simulink model "system13"  (R2019a)
settings: Solver=VariableStepAuto  StartTime=0.0  StopTime=40.0  RelTol=1e-3
values from neighbouring files (symbols this model uses):
  d_y0 = 0    [Lab2.m]
  k2 = sqrt(2*k1)    [Lab2.m]    (also in blockFunc10.m)
  y0 = 0    [Lab2.m]
undefined symbols (not defined in the file or in its folder): sigbuilder_block
settings Model: Creator=Vasco  LastModifiedBy=Vasco

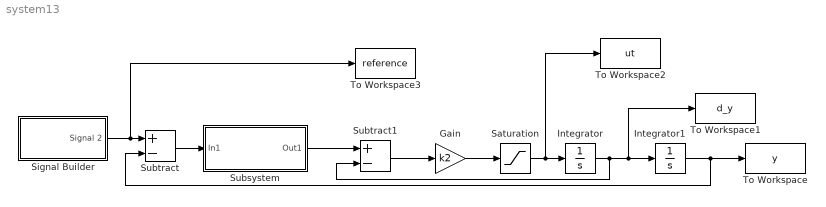
== system system13 ==
  Gain : Gain  Gain=k2
  Integrator : Integrator  InitialCondition=d_y0
  Integrator1 : Integrator  InitialCondition=y0
  Saturation : Saturate  UpperLimit=1  LowerLimit=-1
  Signal Builder : Subsystem  Tag=STV Subsys  LoadFcn=sigbuilder_block('load');  StartFcn=sigbuilder_block('start');  StopFcn=sigbuilder_block('stop');  ClipboardFcn=sigbuilder_block('clipboard');  mask(Sigbuilder block){tuvar=[0:10]}
      mask help: Simulink:masks:SigbuilderBlock_MD
      mask init:
      | if ~strcmp(get_param(bdroot(gcbh),'SimulationStatus'),'stopped') tuvar = sigbuilder_block('maskInit'); end
      settings: CopyFcn=sigbuilder_block('copy');  DeleteFcn=sigbuilder_block('delete');  ModelCloseFcn=sigbuilder_block('modelClose');  PreSaveFcn=sigbuilder_block('preSave');  PauseFcn=sigbuilder_block('pause');  ContinueFcn=sigbuilder_block('continue');  NameChangeFcn=sigbuilder_block('namechange');  OpenFcn=sigbuilder_block('open',[6 30 1012.5 447.75 ]);  CloseFcn=sigbuilder_block('close');
      mask Display: plot(0, 0, 100, 100,[2, 2, 32, 32, 2], [68, 8, 8, 68, 68],[32, 2], [38, 38], [32, 19, 2],[53, 60, 44], [32, 17, 17, 2],[16, 16, 31, 31]);txt = getActiveGroup(gcbh);text(2, 100, txt,'verticalAlignment', 'top');
  Subsystem : Subsystem
  Subtract : Sum  Inputs=+-
  Subtract1 : Sum  Inputs=+-
  To Workspace : ToWorkspace  VariableName=y  SampleTime=-1
      settings: Save2DSignal=2-D array (concatenate along first dimension)
  To Workspace1 : ToWorkspace  VariableName=d_y  SampleTime=-1
      settings: Save2DSignal=2-D array (concatenate along first dimension)
  To Workspace2 : ToWorkspace  VariableName=ut  SampleTime=-1
      settings: Save2DSignal=2-D array (concatenate along first dimension)
  To Workspace3 : ToWorkspace  VariableName=reference  SampleTime=-1
      settings: Save2DSignal=2-D array (concatenate along first dimension)
  wires:
  Subtract1/1 -> Gain/1
  Integrator1/1 -> To Workspace/1, Subtract/2
  Subsystem/1(Out1) -> Subtract1/1
  Subtract/1 -> Subsystem/1(In1)
  Integrator/1 -> Subtract1/2, To Workspace1/1, Integrator1/1
  Gain/1 -> Saturation/1
  Saturation/1 -> To Workspace2/1, Integrator/1
  Signal Builder/1(Signal 2) -> To Workspace3/1, Subtract/1

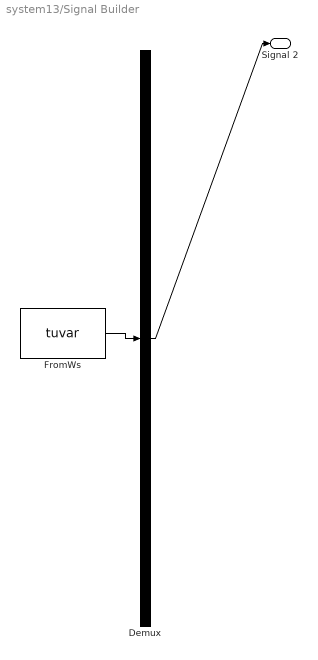
== system system13/Signal Builder ==
  Demux : Demux  Tag=STV Demux  Outputs=1
  FromWs : FromWorkspace  Tag=STV FromWs  VariableName=tuvar  SampleTime=0
      SigBuilderData=|
      | common.afterFinalStr = 'Extrapolate'
      | common.sampleTime = 0
      | dataSet.timeRange = [0 40]
      | dataSet.name = 'Group 1'
      | sbobj.Groups.Name = 'Group 1'
      | sbobj.Groups.Signals.Name = 'Signal 2'
      | sbobj.Groups.Signals.XData = [0 16 24 40]
      | sbobj.Groups.Signals.YData = [4 4 0.98 1.98]
      | sbobj.Groups.TimeRange = [0 40]
  Signal 2 : Outport  Tag=STV Outport
  wires:
  FromWs/1 -> Demux/1
  Demux/1 -> Signal 2/1

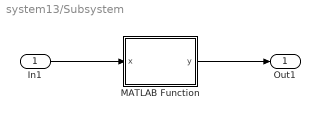
== system system13/Subsystem ==
  In1 : Inport
  MATLAB Function : MATLAB Function  TreatAsAtomicUnit=on
  Out1 : Outport
  wires:
  In1/1 -> MATLAB Function/1(x)
  MATLAB Function/1(y) -> Out1/1

== matlab function system13/Subsystem/MATLAB Function ==
  data: x input; y output
function y = fcn(x)
y1 = 1;
k1 = 1/y1;
k2 = sqrt(2*k1);
    
    if abs(x) <= y1
        y = (k1/k2)*x;
    elseif abs(x) > y1    
        y = sign(x) * (sqrt(2*abs(x))-(1/k2));
    else
        y = 0;
    end

end
